simulink model "control_system_iofbl"  (R2025b)
settings: Solver=FixedStepAuto  StartTime=0.0  StopTime=20  FixedStep=0.01  RelTol=1e-3
values from neighbouring files (symbols this model uses):
  A1 = 0    [init_control_system_iofbl.m]
  A2 = 0    [init_control_system_iofbl.m]
  k = 15    [init_control_system_iofbl.m]
  x0 = [1 1.5]'    [init_control_system_iofbl.m]
  x1d = 2.7081    [init_control_system_iofbl.m]
  x2d = 2.7081    [init_control_system_iofbl.m]
  yd = x1d    (= 2.7081)    [init_control_system_iofbl.m]
libraries: simulink x1
settings Model: Creator=ricca  LastModifiedBy=ricca

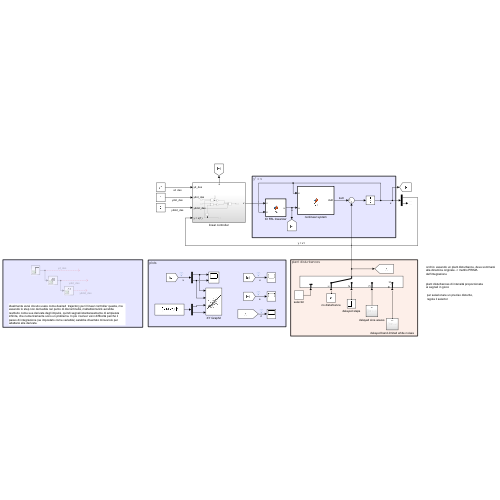
[thumbnail: Simulink's stored preview of the top-level diagram]
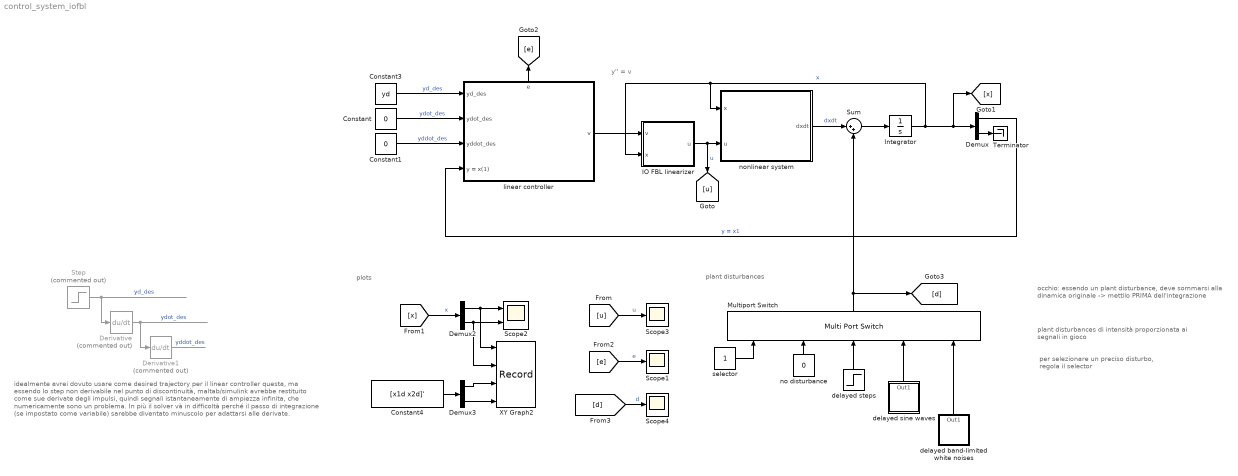
== system control_system_iofbl ==
  note: idealmente avrei dovuto usare come desired trajectory per il linear controller questa, ma essendo lo step non derivabile nel punto di discontinuità, maltab/simulink avrebbe restituito come sue derivate degli impulsi, quindi segnali istantaneamente di ampiezza infinita, che numericamente sono un problema. In più il solver và in difficoltà perché il passo di integrazione (se impostato come variabile) sarebbe diventato minuscolo per adattarsi alle derivate.
  note: y'' = v
  note: plots
  note: plant disturbances
  note: occhio: essendo un plant disturbance, deve sommarsi alla dinamica originale -> mettilo PRIMA dell'integrazione
  note: per selezionare un preciso disturbo, regola il selector
  note: plant disturbances di intensità proporzionata ai segnali in gioco
  Constant : Constant  Value=0
  Constant1 : Constant  Value=0
  Constant3 : Constant  Value=yd
  Constant4 : Constant  Value=[x1d x2d]'
  Demux : Demux  Outputs=2
  Demux2 : Demux  Outputs=2
  Demux3 : Demux  Outputs=2
  Derivative : Derivative  Commented=on
  Derivative1 : Derivative  Commented=on
  IO FBL linearizer : MATLAB Function  TreatAsAtomicUnit=on
  Integrator : Integrator  InitialCondition=x0
  Multiport Switch : MultiPortSwitch  Inputs=4  SaturateOnIntegerOverflow=off  InputSameDT=off
  Scope1 : Scope
      settings: ActiveDisplayYMinimum=-1  ActiveDisplayYMaximum=1
  Scope2 : Scope  NumInputPorts=2
      settings: ActiveDisplayYMinimum=0.59700937630213358  ActiveDisplayYMaximum=4.8921346802383825  DataLoggingVariableName=ScopeData2
  Scope3 : Scope
      settings: ActiveDisplayYMinimum=-1  ActiveDisplayYMaximum=1  DataLoggingVariableName=ScopeData3
  Scope4 : Scope
      settings: ActiveDisplayYMinimum=-1  ActiveDisplayYMaximum=1
  Step : Step  Commented=on  SampleTime=0
  Sum : Sum  Inputs=|++
  Terminator : Terminator
  XY Graph2 : Record  NumPorts=4.0  FileSettingsInternal="{\"entries\":[{\"content\":{\"excelSettings\":{\"content\":{},\"type\":\"Streamout.ExcelSettings\"},\"parquetSettings\":{\"content\":{},\"type\":\"Streamout.ParquetSettings\"}},\"type\":\"Streamout.FileSettingStorage\",\"uuid\":\"\"}],\"packageUris\":[\"http:\\/\\/schema.mathworks.com\\/mf0\\/streamout_blocks\\/R2020a\"],\"version\":\"1.0\"}"  FrameSettings=[0, 0, 0, 0]  Layout=[1 1]  SignalsInternal="{\"entries\":[{\"content\":{\"signals\":[{\"content\":{\"blockPath\":[],\"dimensions\":[1],\"domain\":\"\",\"lineColor\":\"#139fff\",\"plots\":[ 1 ],\"port\":1,\"signalID\":1,\"signalName\":\"Demux2:1\"},\"type\":\"RecordBlkView.Signal\",\"uuid\":\"\"},{\"content\":{\"blockPath\":[],\"dimensions\":[1],\"domain\":\"\",\"lineColor\":\"#139fff\",\"plots\":[ 1 ],\"port\":2,\"signalID\":2,\"signalName\":\"Demux2:2\"},\"type\":\"RecordBlkView.Signal\",\"uuid\":\"\"},{\"content\":{\"blockPath\":[],\"dimensions\":[1],\"domain\":\"\",\"lineColor\":\"#a2142f\",\"lineWidth\":20,\"plots\":[ 1 ],\"port\":3,\"signalID\":3,\"signalName\":\"Demux3:1\"},\"type\":\"RecordBlkView.Signal\",\"uuid\":\"\"},{\"content\":{\"blockPath\":[],\"dimensions\":[1],\"domain\":\"\",\"lineColor\":\"#a2142f\",\"lineWidth\":20,\"plots\":[ 1 ],\"port\":4,\"signalID\":4,\"signalName\":\"Demux3:2\"},\"type\":\"RecordBlkView.Signal\",\"uuid\":\"\"}]},\"type\":\"RecordBlkView.InputSignals\",\"uuid\":\"\"}],\"packageUris\":[\"http:\\/\\/schema.mathworks.com\\/mf0\\/streamout_blocks\\/R2020a\"],\"version\":\"1.0\"}"  VisualizationBindings="{\"xyplotplugin\":{\"info\":[{\"series\":[{\"bindingParametersList\":[{\"parameter\":\"X-Axis\",\"signalID\":3,\"signalName\":\"Demux3:1\"},{\"parameter\":\"Y-Axis\",\"signalID\":4,\"signalName\":\"Demux3:2\"}],\"seriesID\":0},{\"bindingParametersList\":[{\"parameter\":\"X-Axis\",\"signalID\":1,\"signalName\":\"Demux2:1\"},{\"parameter\":\"Y-Axis\",\"signalID\":2,\"signalName\":\"Demux2:2\"}],\"seriesID\":1}],\"subplotID\":1}]}}"  CompatibilityTag=XY
  delayed band-limited white noises : Subsystem
  delayed sine waves : Subsystem
  delayed steps : Step  Time=[7 8]'  After=[0.5 0.6]'  SampleTime=0
  linear controller : Subsystem
      settings: PortSchema="{\"entries\":[{\"content\":{\"sides\":[{\"content\":{\"connectorIds\":[\"In1\",\"In2\",\"In3\",\"In4\"]},\"type\":\"ConnectorPlacement.EquallySpacedRectSide\",\"uuid\":\"bc535d91-cfc4-41be-ae9d-9165ec952d45\"},{\"content\":{\"connectorIds\":[\"Out1\"],\"side\":\"RIGHT\"},\"type\":\"ConnectorPlacement.EquallySpacedRectSide\",\"uuid\":\"7cec438f-9a3b-49c7-ab1c-9bed7e0f3371\"},{\"content\":{\"connectorIds\":[\"Out2\"],\"side\":\"TOP\"},\"type\":\"ConnectorPlacement.EquallySpacedRectSide\",\"uuid\":\"e16798d8-bc2f-4fb9-b582-d3ea06d99f36\"}]},\"type\":\"ConnectorPlacement.EquallySpacedConnector\",\"uuid\":\"e0820c7c-2b09-413a-874c-354f87746b77\"}],\"packageUris\":[\"http://schema.mathworks.com/mf0/Connector/R2020b\"],\"version\":\"1.0\"}"
  no disturbance : Constant  Value=0  OutDataTypeStr=Inherit: Inherit via back propagation
  nonlinear system : MATLAB Function  TreatAsAtomicUnit=on
  selector : Constant
  wires:
  Derivative1/1 -> ?  "yddot_des"
  Constant/1 -> linear controller/2(ydot_des)  "ydot_des"
  Constant1/1 -> linear controller/3(yddot_des)  "yddot_des"
  Step/1 -> Derivative/1  "yd_des"
  Derivative/1 -> Derivative1/1  "ydot_des"
  IO FBL linearizer/1(u) -> [u], nonlinear system/2(u)  "u"
  linear controller/1(v) -> IO FBL linearizer/1(v)
  Constant3/1 -> linear controller/1(yd_des)  "yd_des"
  nonlinear system/1(dxdt) -> Sum/1  "dxdt"
  Demux/1 -> linear controller/4(y = x(1))  "y = x1"
  Demux3/1 -> XY Graph2/3
  Constant4/1 -> Demux3/1
  Demux2/2 -> XY Graph2/2, Scope2/2
  [x] -> Demux2/1  "x"
  Demux3/2 -> XY Graph2/4
  Demux2/1 -> XY Graph2/1, Scope2/1
  [u] -> Scope3/1  "u"
  Demux/2 -> Terminator/1
  Integrator/1 -> [x], Demux/1, IO FBL linearizer/2(x), nonlinear system/1(x)  "x"
  Sum/1 -> Integrator/1
  linear controller/2(e) -> [e]
  [e] -> Scope1/1  "e"
  [d] -> Scope4/1  "d"
  selector/1 -> Multiport Switch/1
  delayed sine waves/1(Out1) -> Multiport Switch/4
  Multiport Switch/1 -> Sum/2, [d]
  no disturbance/1 -> Multiport Switch/2
  delayed band-limited white noises/1(Out1) -> Multiport Switch/5
  delayed steps/1 -> Multiport Switch/3

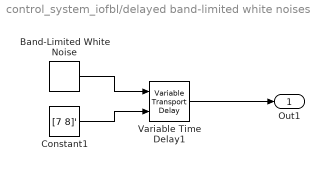
== system control_system_iofbl/delayed band-limited white noises ==
  Band-Limited White Noise : simulink/Sources/Band-Limited White Noise  Cov=[0.01 0.01]'  Ts=0.1  seed=[23341 23342]'
  Constant1 : Constant  Value=[7 8]'
  Variable Time Delay1 : VariableTransportDelay  MaximumDelay=10
  Out1 : Outport
  wires:
  Constant1/1 -> Variable Time Delay1/2
  Band-Limited White Noise/1 -> Variable Time Delay1/1
  Variable Time Delay1/1 -> Out1/1

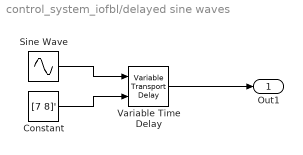
== system control_system_iofbl/delayed sine waves ==
  Constant : Constant  Value=[7 8]'
  Sine Wave : Sin  Amplitude=[0.5 0.6]'  Bias=[0 0]'  SampleTime=0
  Variable Time Delay : VariableTransportDelay  MaximumDelay=10
  Out1 : Outport
  wires:
  Sine Wave/1 -> Variable Time Delay/1
  Variable Time Delay/1 -> Out1/1
  Constant/1 -> Variable Time Delay/2

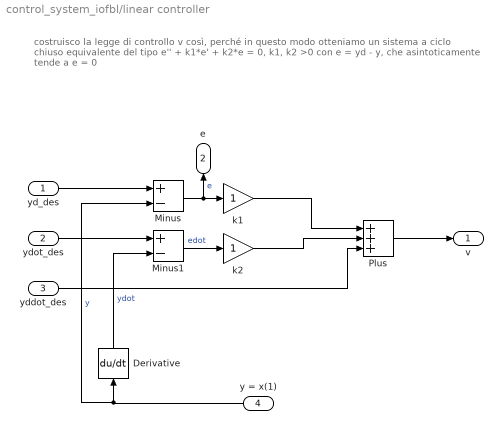
== system control_system_iofbl/linear controller ==
  note: costruisco la legge di controllo v così, perché in questo modo otteniamo un sistema a ciclo chiuso equivalente del tipo
      |
      |                                          e'' + k1*e' + k2*e = 0,          k1, k2 >0
      |
      | con  e = yd - y,  che asintoticamente tende a e = 0
  yd_des : Inport
  ydot_des : Inport  Port=2
  yddot_des : Inport  Port=3
  y = x(1) : Inport  Port=4
  Derivative : Derivative
  Minus : Sum  Inputs=+-
  Minus1 : Sum  Inputs=+-
  Plus : Sum  Inputs=+++
  k1 : Gain
  k2 : Gain
  v : Outport
  e : Outport  Port=2
  wires:
  Derivative/1 -> Minus1/2  "ydot"
  y = x(1)/1 -> Derivative/1, Minus/2  "y"
  k2/1 -> Plus/2
  yd_des/1 -> Minus/1
  Minus1/1 -> k2/1  "edot"
  k1/1 -> Plus/1
  Minus/1 -> e/1, k1/1  "e"
  ydot_des/1 -> Minus1/1
  Plus/1 -> v/1
  yddot_des/1 -> Plus/3

== matlab function control_system_iofbl/IO FBL linearizer ==
  data: v input; u output; x input; A1 parameter; A2 parameter; k parameter
function u = fcn(v,x,A1, A2, k)

% l1 e l2 sono copiati e incollati dal file matlab associato

l1 = -k*exp(-x(2))*(x(2) - 1);
l2 = x(1) - A1 - k*x(2)*exp(-x(2)) - k*exp(-x(2))*(x(2) - 1)*(A2 - x(2) + k*x(1)*exp(-x(1)));
u = (1/l1)*(-l2 + v);

end

== matlab function control_system_iofbl/nonlinear system ==
  data: x input; u input; dxdt output; A1 parameter; A2 parameter; k parameter
function dxdt = fcn(x,u,A1, A2, k)

dxdt = [-x(1) + A2 + k*x(2)*exp(-x(2));           
        -x(2) + A1 + k*x(1)*exp(-x(1)) + u];    

%% se vuoi testare la sensibilità rispetto a unmodelled dynamics  Delta_f, uncommmenta i Delta_f e dxdt sotto, e commmenta il dxdt sopra.

% Delta_f = 0.2*sin(x(1));
% dxdt = [-x(1) + A2 + k*x(2)*exp(-x(2)) + Delta_f;           
%         -x(2) + A1 + k*x(1)*exp(-x(1)) + Delta_f + u];    

%% se vuoi testare la sensibilità rispetto a parametric uncertainties del 10% su k, uncommmenta dxdt sotto, e commmenta il dxdt sopra.

% dxdt = [-x(1) + A2 + (k+0.10*k)*x(2)*exp(-x(2));           
%         -x(2) + A1 + (k+0.10*k)*x(1)*exp(-x(1)) + u];    
  

end
